simulink library "sub_lib_models"  (Simulink 4.00)
undefined symbols (not defined in the file or in its folder): vinf
libraries: lib_cosimulation x22
settings Model: LastModifiedBy=abrooker
settings Model: ModifiedComment=|
  | abrooker -- Thu May 02 17:18:54 2002 -- Version 1.26
  | fixed starter load level for non-cosim runs
settings Model: ModifiedHistory=|
  | abrooker -- Thu May 02 17:18:54 2002 -- Version 1.26
  | fixed starter load level for non-cosim runs
  | 
  | abrooker -- Wed Apr 24 09:14:19 2002 -- Version 1.25
  | 
  | 
  | abrooker -- Fri Apr 19 08:51:04 2002 -- Version 1.24
  | 
  | 
  | abrooker -- Fri Apr 19 08:49:53 2002 -- Version 1.23
  | 
  | 
  | mokeefe -- Thu Apr 18 08:41:06 2002 -- Version 1.22
  | saving the model:
  | o "without the model browser open"
  | o with only top-level screen visible
  | o with "fit to view" enabled
  | o with "status bar" off and "toolbar" off
  | o with "prompt to update model history with each save" on

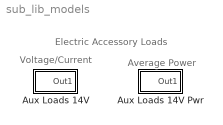
== system sub_lib_models ==
  note: Electric Accessory Loads
  note: Voltage/Current
  note: Average Power
  Aux Loads 14V : Subsystem
      settings: RTWFcnNameOpts=Auto  RTWFileNameOpts=Auto
  Aux Loads 14V Pwr : Subsystem
      settings: RTWFcnNameOpts=Auto  RTWFileNameOpts=Auto

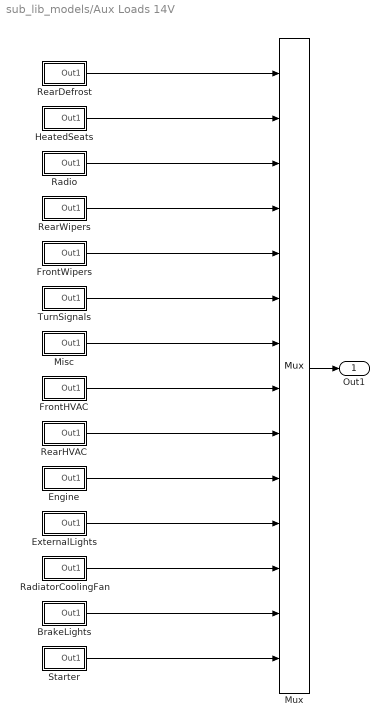
== system sub_lib_models/Aux Loads 14V ==
  BrakeLights : Subsystem
      settings: RTWFcnNameOpts=Auto  RTWFileNameOpts=Auto
  Engine : Subsystem
      settings: RTWFcnNameOpts=Auto  RTWFileNameOpts=Auto
  ExternalLights : Subsystem
      settings: RTWFcnNameOpts=Auto  RTWFileNameOpts=Auto
  FrontHVAC : Subsystem
      settings: RTWFcnNameOpts=Auto  RTWFileNameOpts=Auto
  FrontWipers : Subsystem
      settings: RTWFcnNameOpts=Auto  RTWFileNameOpts=Auto
  HeatedSeats : Subsystem
      settings: RTWFcnNameOpts=Auto  RTWFileNameOpts=Auto
  Misc : Subsystem
      settings: RTWFcnNameOpts=Auto  RTWFileNameOpts=Auto
  Mux : Mux  Inputs=[8 9 8 8 8 8 8 9 9 8 9 9 8 2]
      settings: DisplayOption=none
  RadiatorCoolingFan : Subsystem
      settings: RTWFcnNameOpts=Auto  RTWFileNameOpts=Auto
  Radio : Subsystem
      settings: RTWFcnNameOpts=Auto  RTWFileNameOpts=Auto
  RearDefrost : Subsystem
      settings: RTWFcnNameOpts=Auto  RTWFileNameOpts=Auto
  RearHVAC : Subsystem
      settings: RTWFcnNameOpts=Auto  RTWFileNameOpts=Auto
  RearWipers : Subsystem
      settings: RTWFcnNameOpts=Auto  RTWFileNameOpts=Auto
  Starter : Subsystem
      settings: RTWFcnNameOpts=Auto  RTWFileNameOpts=Auto
  TurnSignals : Subsystem
      settings: RTWFcnNameOpts=Auto  RTWFileNameOpts=Auto
  Out1 : Outport  Port=1
  wires:
  Starter/1(Out1) -> Mux/14
  BrakeLights/1(Out1) -> Mux/13
  RadiatorCoolingFan/1(Out1) -> Mux/12
  ExternalLights/1(Out1) -> Mux/11
  Engine/1(Out1) -> Mux/10
  RearHVAC/1(Out1) -> Mux/9
  FrontHVAC/1(Out1) -> Mux/8
  Misc/1(Out1) -> Mux/7
  TurnSignals/1(Out1) -> Mux/6
  FrontWipers/1(Out1) -> Mux/5
  RearWipers/1(Out1) -> Mux/4
  Radio/1(Out1) -> Mux/3
  HeatedSeats/1(Out1) -> Mux/2
  RearDefrost/1(Out1) -> Mux/1
  Mux/1 -> Out1/1

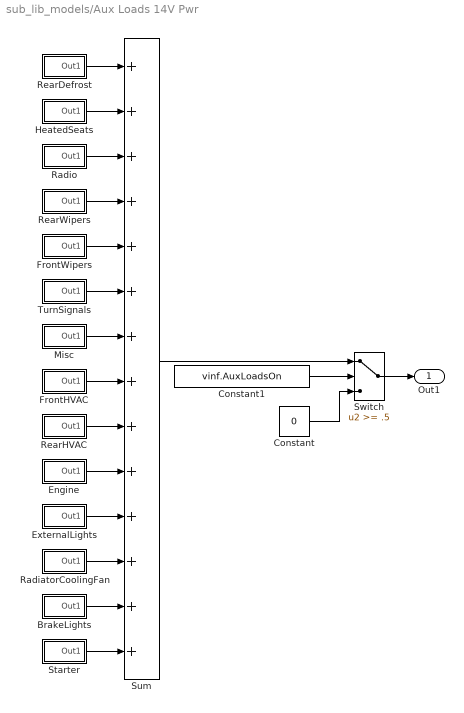
== system sub_lib_models/Aux Loads 14V Pwr ==
  BrakeLights : Subsystem
      settings: RTWFcnNameOpts=Auto  RTWFileNameOpts=Auto
  Constant : Constant  Value=0
  Constant1 : Constant  Value=vinf.AuxLoadsOn
  Engine : Subsystem
      settings: RTWFcnNameOpts=Auto  RTWFileNameOpts=Auto
  ExternalLights : Subsystem
      settings: RTWFcnNameOpts=Auto  RTWFileNameOpts=Auto
  FrontHVAC : Subsystem
      settings: RTWFcnNameOpts=Auto  RTWFileNameOpts=Auto
  FrontWipers : Subsystem
      settings: RTWFcnNameOpts=Auto  RTWFileNameOpts=Auto
  HeatedSeats : Subsystem
      settings: RTWFcnNameOpts=Auto  RTWFileNameOpts=Auto
  Misc : Subsystem
      settings: RTWFcnNameOpts=Auto  RTWFileNameOpts=Auto
  RadiatorCoolingFan : Subsystem
      settings: RTWFcnNameOpts=Auto  RTWFileNameOpts=Auto
  Radio : Subsystem
      settings: RTWFcnNameOpts=Auto  RTWFileNameOpts=Auto
  RearDefrost : Subsystem
      settings: RTWFcnNameOpts=Auto  RTWFileNameOpts=Auto
  RearHVAC : Subsystem
      settings: RTWFcnNameOpts=Auto  RTWFileNameOpts=Auto
  RearWipers : Subsystem
      settings: RTWFcnNameOpts=Auto  RTWFileNameOpts=Auto
  Starter : Subsystem
      settings: RTWFcnNameOpts=Auto  RTWFileNameOpts=Auto
  Sum : Sum  Inputs=++++++++++++++  SaturateOnIntegerOverflow=on
  Switch : Switch  Threshold=.5
  TurnSignals : Subsystem
      settings: RTWFcnNameOpts=Auto  RTWFileNameOpts=Auto
  Out1 : Outport  Port=1
  wires:
  Switch/1 -> Out1/1
  Sum/1 -> Switch/1
  Constant/1 -> Switch/3
  Constant1/1 -> Switch/2
  RearDefrost/1(Out1) -> Sum/1
  HeatedSeats/1(Out1) -> Sum/2
  Radio/1(Out1) -> Sum/3
  RearWipers/1(Out1) -> Sum/4
  FrontWipers/1(Out1) -> Sum/5
  TurnSignals/1(Out1) -> Sum/6
  Misc/1(Out1) -> Sum/7
  FrontHVAC/1(Out1) -> Sum/8
  RearHVAC/1(Out1) -> Sum/9
  Engine/1(Out1) -> Sum/10
  ExternalLights/1(Out1) -> Sum/11
  RadiatorCoolingFan/1(Out1) -> Sum/12
  BrakeLights/1(Out1) -> Sum/13
  Starter/1(Out1) -> Sum/14

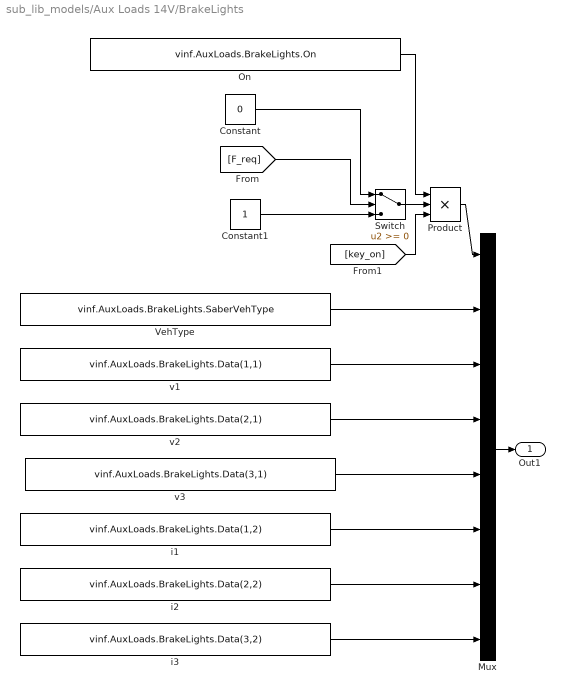
== system sub_lib_models/Aux Loads 14V/BrakeLights ==
  Constant : Constant  Value=0
  Constant1 : Constant  Value=1
  Mux : Mux  Inputs=8
  On : Constant  Value=vinf.AuxLoads.BrakeLights.On
  Product : Product  Inputs=3  Multiplication=Element-wise(.*)  SaturateOnIntegerOverflow=on
  Switch : Switch  Threshold=0
  VehType : Constant  Value=vinf.AuxLoads.BrakeLights.SaberVehType
  i1 : Constant  Value=vinf.AuxLoads.BrakeLights.Data(1,2)
  i2 : Constant  Value=vinf.AuxLoads.BrakeLights.Data(2,2)
  i3 : Constant  Value=vinf.AuxLoads.BrakeLights.Data(3,2)
  v1 : Constant  Value=vinf.AuxLoads.BrakeLights.Data(1,1)
  v2 : Constant  Value=vinf.AuxLoads.BrakeLights.Data(2,1)
  v3 : Constant  Value=vinf.AuxLoads.BrakeLights.Data(3,1)
  Out1 : Outport  Port=1
  wires:
  [key_on] -> Product/3
  VehType/1 -> Mux/2
  i3/1 -> Mux/8
  i2/1 -> Mux/7
  i1/1 -> Mux/6
  v3/1 -> Mux/5
  v2/1 -> Mux/4
  v1/1 -> Mux/3
  Mux/1 -> Out1/1
  On/1 -> Product/1
  Product/1 -> Mux/1
  Constant/1 -> Switch/1
  [F_req] -> Switch/2
  Constant1/1 -> Switch/3
  Switch/1 -> Product/2

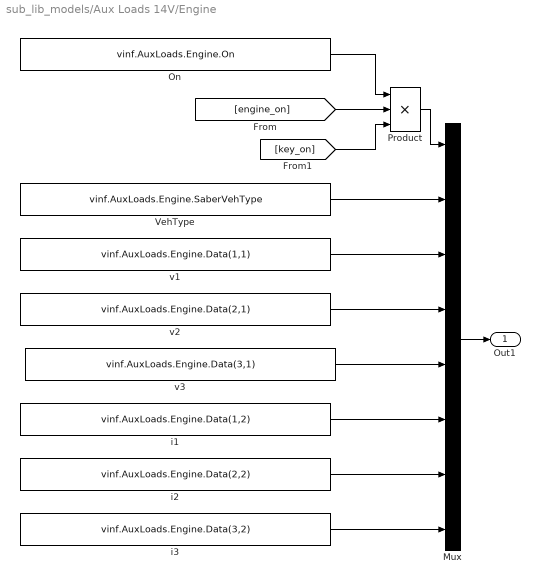
== system sub_lib_models/Aux Loads 14V/Engine ==
  Mux : Mux  Inputs=8
  On : Constant  Value=vinf.AuxLoads.Engine.On
  Product : Product  Inputs=3  Multiplication=Element-wise(.*)  SaturateOnIntegerOverflow=on
  VehType : Constant  Value=vinf.AuxLoads.Engine.SaberVehType
  i1 : Constant  Value=vinf.AuxLoads.Engine.Data(1,2)
  i2 : Constant  Value=vinf.AuxLoads.Engine.Data(2,2)
  i3 : Constant  Value=vinf.AuxLoads.Engine.Data(3,2)
  v1 : Constant  Value=vinf.AuxLoads.Engine.Data(1,1)
  v2 : Constant  Value=vinf.AuxLoads.Engine.Data(2,1)
  v3 : Constant  Value=vinf.AuxLoads.Engine.Data(3,1)
  Out1 : Outport  Port=1
  wires:
  [key_on] -> Product/3
  i3/1 -> Mux/8
  i2/1 -> Mux/7
  i1/1 -> Mux/6
  v3/1 -> Mux/5
  v2/1 -> Mux/4
  v1/1 -> Mux/3
  Mux/1 -> Out1/1
  On/1 -> Product/1
  [engine_on] -> Product/2
  Product/1 -> Mux/1
  VehType/1 -> Mux/2

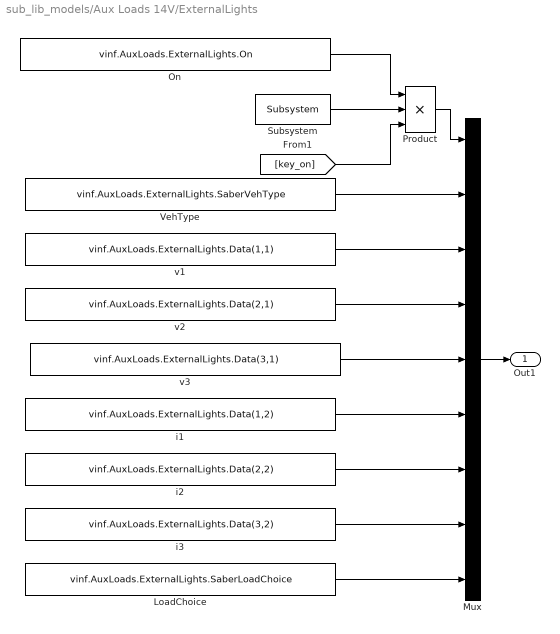
== system sub_lib_models/Aux Loads 14V/ExternalLights ==
  LoadChoice : Constant  Value=vinf.AuxLoads.ExternalLights.SaberLoadChoice
  Mux : Mux  Inputs=9
  On : Constant  Value=vinf.AuxLoads.ExternalLights.On
  Product : Product  Inputs=3  Multiplication=Element-wise(.*)  SaturateOnIntegerOverflow=on
  Subsystem : lib_cosimulation/Subsystem  ModelName='ExternalLights'
  VehType : Constant  Value=vinf.AuxLoads.ExternalLights.SaberVehType
  i1 : Constant  Value=vinf.AuxLoads.ExternalLights.Data(1,2)
  i2 : Constant  Value=vinf.AuxLoads.ExternalLights.Data(2,2)
  i3 : Constant  Value=vinf.AuxLoads.ExternalLights.Data(3,2)
  v1 : Constant  Value=vinf.AuxLoads.ExternalLights.Data(1,1)
  v2 : Constant  Value=vinf.AuxLoads.ExternalLights.Data(2,1)
  v3 : Constant  Value=vinf.AuxLoads.ExternalLights.Data(3,1)
  Out1 : Outport  Port=1
  wires:
  [key_on] -> Product/3
  LoadChoice/1 -> Mux/9
  i3/1 -> Mux/8
  i2/1 -> Mux/7
  i1/1 -> Mux/6
  v3/1 -> Mux/5
  v2/1 -> Mux/4
  v1/1 -> Mux/3
  VehType/1 -> Mux/2
  Mux/1 -> Out1/1
  On/1 -> Product/1
  Subsystem/1 -> Product/2
  Product/1 -> Mux/1

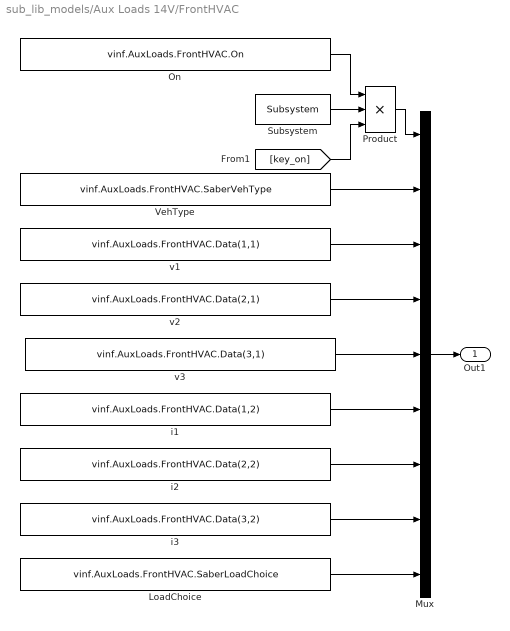
== system sub_lib_models/Aux Loads 14V/FrontHVAC ==
  LoadChoice : Constant  Value=vinf.AuxLoads.FrontHVAC.SaberLoadChoice
  Mux : Mux  Inputs=9
  On : Constant  Value=vinf.AuxLoads.FrontHVAC.On
  Product : Product  Inputs=3  Multiplication=Element-wise(.*)  SaturateOnIntegerOverflow=on
  Subsystem : lib_cosimulation/Subsystem  ModelName='FrontHVAC'
  VehType : Constant  Value=vinf.AuxLoads.FrontHVAC.SaberVehType
  i1 : Constant  Value=vinf.AuxLoads.FrontHVAC.Data(1,2)
  i2 : Constant  Value=vinf.AuxLoads.FrontHVAC.Data(2,2)
  i3 : Constant  Value=vinf.AuxLoads.FrontHVAC.Data(3,2)
  v1 : Constant  Value=vinf.AuxLoads.FrontHVAC.Data(1,1)
  v2 : Constant  Value=vinf.AuxLoads.FrontHVAC.Data(2,1)
  v3 : Constant  Value=vinf.AuxLoads.FrontHVAC.Data(3,1)
  Out1 : Outport  Port=1
  wires:
  [key_on] -> Product/3
  LoadChoice/1 -> Mux/9
  i3/1 -> Mux/8
  i2/1 -> Mux/7
  i1/1 -> Mux/6
  v3/1 -> Mux/5
  v2/1 -> Mux/4
  v1/1 -> Mux/3
  VehType/1 -> Mux/2
  Mux/1 -> Out1/1
  On/1 -> Product/1
  Subsystem/1 -> Product/2
  Product/1 -> Mux/1

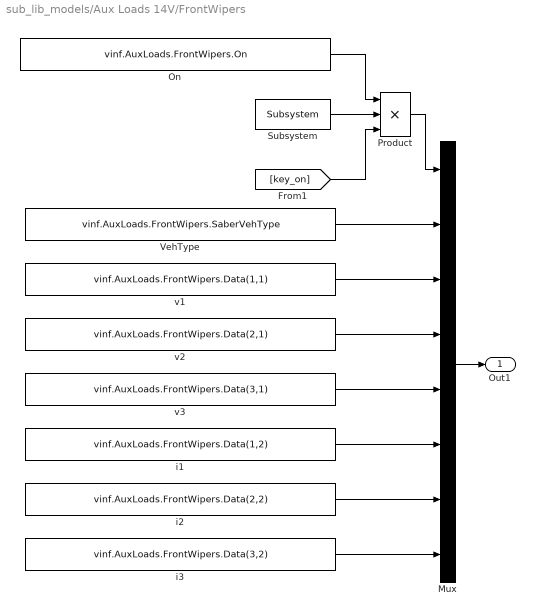
== system sub_lib_models/Aux Loads 14V/FrontWipers ==
  Mux : Mux  Inputs=8
  On : Constant  Value=vinf.AuxLoads.FrontWipers.On
  Product : Product  Inputs=3  Multiplication=Element-wise(.*)  SaturateOnIntegerOverflow=on
  Subsystem : lib_cosimulation/Subsystem  ModelName='FrontWipers'
  VehType : Constant  Value=vinf.AuxLoads.FrontWipers.SaberVehType
  i1 : Constant  Value=vinf.AuxLoads.FrontWipers.Data(1,2)
  i2 : Constant  Value=vinf.AuxLoads.FrontWipers.Data(2,2)
  i3 : Constant  Value=vinf.AuxLoads.FrontWipers.Data(3,2)
  v1 : Constant  Value=vinf.AuxLoads.FrontWipers.Data(1,1)
  v2 : Constant  Value=vinf.AuxLoads.FrontWipers.Data(2,1)
  v3 : Constant  Value=vinf.AuxLoads.FrontWipers.Data(3,1)
  Out1 : Outport  Port=1
  wires:
  [key_on] -> Product/3
  VehType/1 -> Mux/2
  i2/1 -> Mux/7
  i3/1 -> Mux/8
  i1/1 -> Mux/6
  v3/1 -> Mux/5
  v2/1 -> Mux/4
  v1/1 -> Mux/3
  Mux/1 -> Out1/1
  On/1 -> Product/1
  Subsystem/1 -> Product/2
  Product/1 -> Mux/1

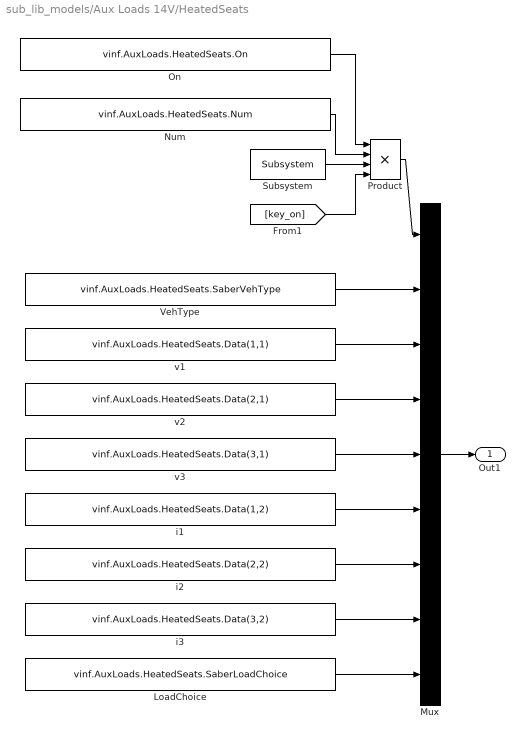
== system sub_lib_models/Aux Loads 14V/HeatedSeats ==
  LoadChoice : Constant  Value=vinf.AuxLoads.HeatedSeats.SaberLoadChoice
  Mux : Mux  Inputs=9
  Num : Constant  Value=vinf.AuxLoads.HeatedSeats.Num
  On : Constant  Value=vinf.AuxLoads.HeatedSeats.On
  Product : Product  Inputs=4  Multiplication=Element-wise(.*)  SaturateOnIntegerOverflow=on
  Subsystem : lib_cosimulation/Subsystem  ModelName='HeatedSeats'
  VehType : Constant  Value=vinf.AuxLoads.HeatedSeats.SaberVehType
  i1 : Constant  Value=vinf.AuxLoads.HeatedSeats.Data(1,2)
  i2 : Constant  Value=vinf.AuxLoads.HeatedSeats.Data(2,2)
  i3 : Constant  Value=vinf.AuxLoads.HeatedSeats.Data(3,2)
  v1 : Constant  Value=vinf.AuxLoads.HeatedSeats.Data(1,1)
  v2 : Constant  Value=vinf.AuxLoads.HeatedSeats.Data(2,1)
  v3 : Constant  Value=vinf.AuxLoads.HeatedSeats.Data(3,1)
  Out1 : Outport  Port=1
  wires:
  Product/1 -> Mux/1
  [key_on] -> Product/4
  Mux/1 -> Out1/1
  LoadChoice/1 -> Mux/9
  v1/1 -> Mux/3
  v2/1 -> Mux/4
  v3/1 -> Mux/5
  i1/1 -> Mux/6
  i2/1 -> Mux/7
  i3/1 -> Mux/8
  VehType/1 -> Mux/2
  On/1 -> Product/1
  Num/1 -> Product/2
  Subsystem/1 -> Product/3

== system sub_lib_models/Aux Loads 14V/Misc ==
  Mux : Mux  Inputs=8
  On : Constant  Value=vinf.AuxLoads.Misc.On
  Product : Product  Inputs=2  Multiplication=Element-wise(.*)  SaturateOnIntegerOverflow=on
  VehType : Constant  Value=vinf.AuxLoads.Misc.SaberVehType
  i1 : Constant  Value=vinf.AuxLoads.Misc.Data(1,2)
  i2 : Constant  Value=vinf.AuxLoads.Misc.Data(2,2)
  i3 : Constant  Value=vinf.AuxLoads.Misc.Data(3,2)
  v1 : Constant  Value=vinf.AuxLoads.Misc.Data(1,1)
  v2 : Constant  Value=vinf.AuxLoads.Misc.Data(2,1)
  v3 : Constant  Value=vinf.AuxLoads.Misc.Data(3,1)
  Out1 : Outport  Port=1
  wires:
  [key_on] -> Product/2
  On/1 -> Product/1
  Product/1 -> Mux/1
  VehType/1 -> Mux/2
  i3/1 -> Mux/8
  i2/1 -> Mux/7
  i1/1 -> Mux/6
  v3/1 -> Mux/5
  v2/1 -> Mux/4
  v1/1 -> Mux/3
  Mux/1 -> Out1/1

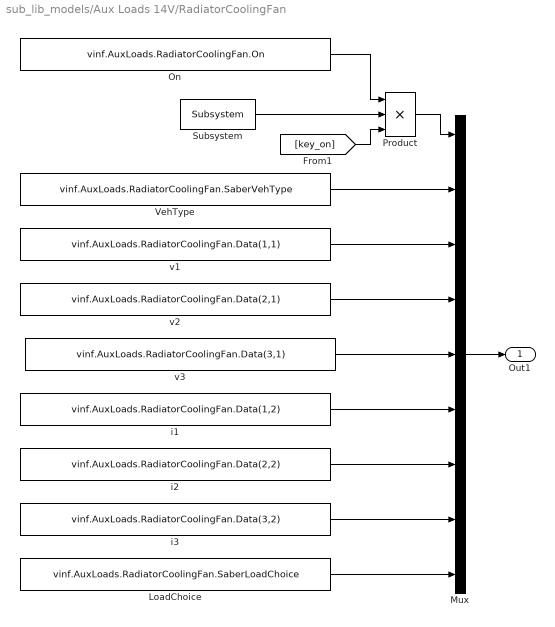
== system sub_lib_models/Aux Loads 14V/RadiatorCoolingFan ==
  LoadChoice : Constant  Value=vinf.AuxLoads.RadiatorCoolingFan.SaberLoadChoice
  Mux : Mux  Inputs=9
  On : Constant  Value=vinf.AuxLoads.RadiatorCoolingFan.On
  Product : Product  Inputs=3  Multiplication=Element-wise(.*)  SaturateOnIntegerOverflow=on
  Subsystem : lib_cosimulation/Subsystem  ModelName='RadiatorCoolingFan'
  VehType : Constant  Value=vinf.AuxLoads.RadiatorCoolingFan.SaberVehType
  i1 : Constant  Value=vinf.AuxLoads.RadiatorCoolingFan.Data(1,2)
  i2 : Constant  Value=vinf.AuxLoads.RadiatorCoolingFan.Data(2,2)
  i3 : Constant  Value=vinf.AuxLoads.RadiatorCoolingFan.Data(3,2)
  v1 : Constant  Value=vinf.AuxLoads.RadiatorCoolingFan.Data(1,1)
  v2 : Constant  Value=vinf.AuxLoads.RadiatorCoolingFan.Data(2,1)
  v3 : Constant  Value=vinf.AuxLoads.RadiatorCoolingFan.Data(3,1)
  Out1 : Outport  Port=1
  wires:
  [key_on] -> Product/3
  Mux/1 -> Out1/1
  LoadChoice/1 -> Mux/9
  i3/1 -> Mux/8
  i2/1 -> Mux/7
  i1/1 -> Mux/6
  v3/1 -> Mux/5
  v2/1 -> Mux/4
  v1/1 -> Mux/3
  VehType/1 -> Mux/2
  On/1 -> Product/1
  Subsystem/1 -> Product/2
  Product/1 -> Mux/1

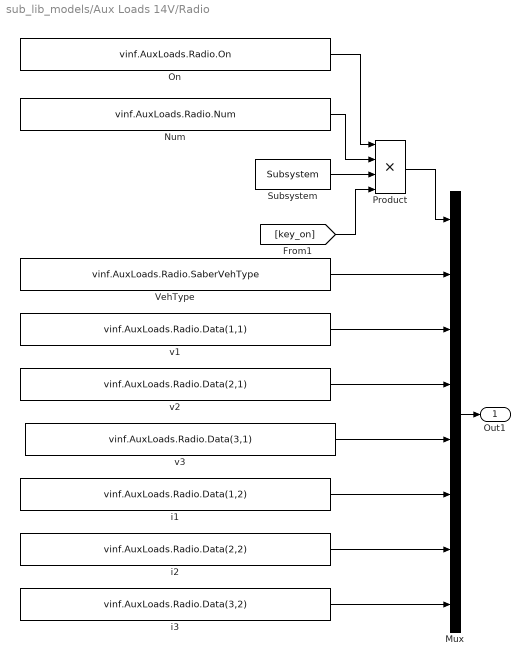
== system sub_lib_models/Aux Loads 14V/Radio ==
  Mux : Mux  Inputs=8
  Num : Constant  Value=vinf.AuxLoads.Radio.Num
  On : Constant  Value=vinf.AuxLoads.Radio.On
  Product : Product  Inputs=4  Multiplication=Element-wise(.*)  SaturateOnIntegerOverflow=on
  Subsystem : lib_cosimulation/Subsystem  ModelName='Radio'
  VehType : Constant  Value=vinf.AuxLoads.Radio.SaberVehType
  i1 : Constant  Value=vinf.AuxLoads.Radio.Data(1,2)
  i2 : Constant  Value=vinf.AuxLoads.Radio.Data(2,2)
  i3 : Constant  Value=vinf.AuxLoads.Radio.Data(3,2)
  v1 : Constant  Value=vinf.AuxLoads.Radio.Data(1,1)
  v2 : Constant  Value=vinf.AuxLoads.Radio.Data(2,1)
  v3 : Constant  Value=vinf.AuxLoads.Radio.Data(3,1)
  Out1 : Outport  Port=1
  wires:
  [key_on] -> Product/4
  i3/1 -> Mux/8
  i2/1 -> Mux/7
  i1/1 -> Mux/6
  v3/1 -> Mux/5
  v2/1 -> Mux/4
  v1/1 -> Mux/3
  VehType/1 -> Mux/2
  Mux/1 -> Out1/1
  On/1 -> Product/1
  Num/1 -> Product/2
  Subsystem/1 -> Product/3
  Product/1 -> Mux/1

== system sub_lib_models/Aux Loads 14V/RearDefrost ==
  Mux : Mux  Inputs=8
  On : Constant  Value=vinf.AuxLoads.RearDefrost.On
  Product : Product  Inputs=3  Multiplication=Element-wise(.*)  SaturateOnIntegerOverflow=on
  Subsystem : lib_cosimulation/Subsystem  ModelName='RearDefrost'
  VehType : Constant  Value=vinf.AuxLoads.RearDefrost.SaberVehType
  i1 : Constant  Value=vinf.AuxLoads.RearDefrost.Data(1,2)
  i2 : Constant  Value=vinf.AuxLoads.RearDefrost.Data(2,2)
  i3 : Constant  Value=vinf.AuxLoads.RearDefrost.Data(3,2)
  v1 : Constant  Value=vinf.AuxLoads.RearDefrost.Data(1,1)
  v2 : Constant  Value=vinf.AuxLoads.RearDefrost.Data(2,1)
  v3 : Constant  Value=vinf.AuxLoads.RearDefrost.Data(3,1)
  Out1 : Outport  Port=1
  wires:
  On/1 -> Product/1
  Subsystem/1 -> Product/2
  [key_on] -> Product/3
  Product/1 -> Mux/1
  VehType/1 -> Mux/2
  i3/1 -> Mux/8
  i2/1 -> Mux/7
  i1/1 -> Mux/6
  v3/1 -> Mux/5
  v2/1 -> Mux/4
  v1/1 -> Mux/3
  Mux/1 -> Out1/1

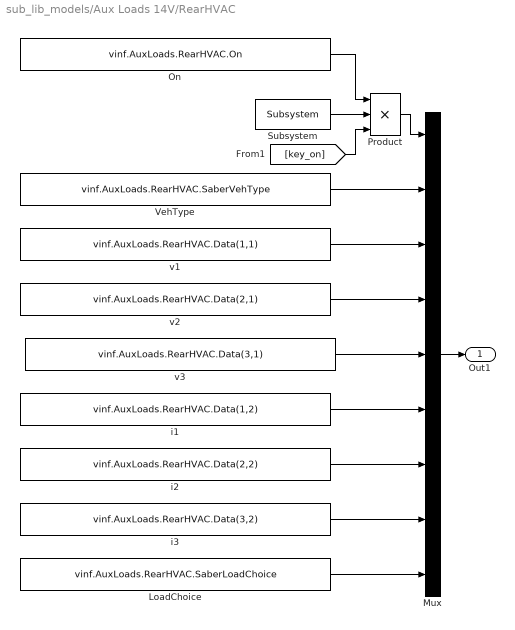
== system sub_lib_models/Aux Loads 14V/RearHVAC ==
  LoadChoice : Constant  Value=vinf.AuxLoads.RearHVAC.SaberLoadChoice
  Mux : Mux  Inputs=9
  On : Constant  Value=vinf.AuxLoads.RearHVAC.On
  Product : Product  Inputs=3  Multiplication=Element-wise(.*)  SaturateOnIntegerOverflow=on
  Subsystem : lib_cosimulation/Subsystem  ModelName='RearHVAC'
  VehType : Constant  Value=vinf.AuxLoads.RearHVAC.SaberVehType
  i1 : Constant  Value=vinf.AuxLoads.RearHVAC.Data(1,2)
  i2 : Constant  Value=vinf.AuxLoads.RearHVAC.Data(2,2)
  i3 : Constant  Value=vinf.AuxLoads.RearHVAC.Data(3,2)
  v1 : Constant  Value=vinf.AuxLoads.RearHVAC.Data(1,1)
  v2 : Constant  Value=vinf.AuxLoads.RearHVAC.Data(2,1)
  v3 : Constant  Value=vinf.AuxLoads.RearHVAC.Data(3,1)
  Out1 : Outport  Port=1
  wires:
  [key_on] -> Product/3
  LoadChoice/1 -> Mux/9
  i3/1 -> Mux/8
  i2/1 -> Mux/7
  i1/1 -> Mux/6
  v3/1 -> Mux/5
  v2/1 -> Mux/4
  v1/1 -> Mux/3
  Mux/1 -> Out1/1
  On/1 -> Product/1
  Subsystem/1 -> Product/2
  Product/1 -> Mux/1
  VehType/1 -> Mux/2

== system sub_lib_models/Aux Loads 14V/RearWipers ==
  Mux : Mux  Inputs=8
  On : Constant  Value=vinf.AuxLoads.RearWipers.On
  Product : Product  Inputs=3  Multiplication=Element-wise(.*)  SaturateOnIntegerOverflow=on
  Subsystem : lib_cosimulation/Subsystem  ModelName='RearWipers'
  VehType : Constant  Value=vinf.AuxLoads.RearWipers.SaberVehType
  i1 : Constant  Value=vinf.AuxLoads.RearWipers.Data(1,2)
  i2 : Constant  Value=vinf.AuxLoads.RearWipers.Data(2,2)
  i3 : Constant  Value=vinf.AuxLoads.RearWipers.Data(3,2)
  v1 : Constant  Value=vinf.AuxLoads.RearWipers.Data(1,1)
  v2 : Constant  Value=vinf.AuxLoads.RearWipers.Data(2,1)
  v3 : Constant  Value=vinf.AuxLoads.RearWipers.Data(3,1)
  Out1 : Outport  Port=1
  wires:
  [key_on] -> Product/3
  i3/1 -> Mux/8
  i2/1 -> Mux/7
  i1/1 -> Mux/6
  v3/1 -> Mux/5
  v2/1 -> Mux/4
  v1/1 -> Mux/3
  Mux/1 -> Out1/1
  On/1 -> Product/1
  Subsystem/1 -> Product/2
  Product/1 -> Mux/1
  VehType/1 -> Mux/2

== system sub_lib_models/Aux Loads 14V/Starter ==
  14 V : Constant  Value=vinf.AuxLoads.Starter.V14
  Hit  Crossing : HitCross  HitCrossingOffset=0  HitCrossingDirection=rising  ShowOutputPort=on
  Mux : Mux  Inputs=2
  On : Constant  Value=vinf.AuxLoads.Starter.On
  Product1 : Product  Inputs=4  Multiplication=Element-wise(.*)  SaturateOnIntegerOverflow=on
  Subsystem : lib_cosimulation/14V Load Control/Starter/Subsystem
      settings: RTWFcnNameOpts=Auto  RTWFileNameOpts=Auto
  starter_load (power) : Constant  Value=vinf.AuxLoads.Starter.Data
  Out1 : Outport  Port=1
  wires:
  Mux/1 -> Out1/1
  starter_load (power)/1 -> Mux/2
  14 V/1 -> Product1/2
  Subsystem/1 -> Product1/3
  Product1/1 -> Mux/1
  On/1 -> Product1/1
  [key_on] -> Product1/4
  [time] -> Subsystem/2
  [engine_on] -> Hit  Crossing/1
  Hit  Crossing/1 -> Subsystem/1

== system sub_lib_models/Aux Loads 14V/TurnSignals ==
  Mux : Mux  Inputs=8
  On : Constant  Value=vinf.AuxLoads.TurnSignals.On
  Product : Product  Inputs=3  Multiplication=Element-wise(.*)  SaturateOnIntegerOverflow=on
  Subsystem : lib_cosimulation/Subsystem  ModelName='TurnSignals'
  VehType : Constant  Value=vinf.AuxLoads.TurnSignals.SaberVehType
  i1 : Constant  Value=vinf.AuxLoads.TurnSignals.Data(1,2)
  i2 : Constant  Value=vinf.AuxLoads.TurnSignals.Data(2,2)
  i3 : Constant  Value=vinf.AuxLoads.TurnSignals.Data(3,2)
  v1 : Constant  Value=vinf.AuxLoads.TurnSignals.Data(1,1)
  v2 : Constant  Value=vinf.AuxLoads.TurnSignals.Data(2,1)
  v3 : Constant  Value=vinf.AuxLoads.TurnSignals.Data(3,1)
  Out1 : Outport  Port=1
  wires:
  [key_on] -> Product/3
  i3/1 -> Mux/8
  i2/1 -> Mux/7
  i1/1 -> Mux/6
  v3/1 -> Mux/5
  v2/1 -> Mux/4
  v1/1 -> Mux/3
  Mux/1 -> Out1/1
  On/1 -> Product/1
  Subsystem/1 -> Product/2
  Product/1 -> Mux/1
  VehType/1 -> Mux/2

== system sub_lib_models/Aux Loads 14V Pwr/BrakeLights ==
  Average Watts : Constant  Value=vinf.AuxLoads.BrakeLights.AverageWatts
  Constant : Constant  Value=0
  Constant1 : Constant  Value=1
  On : Constant  Value=vinf.AuxLoads.BrakeLights.On
  Product : Product  Inputs=4  Multiplication=Element-wise(.*)  SaturateOnIntegerOverflow=on
  Switch : Switch  Threshold=0
  Out1 : Outport  Port=1
  wires:
  Switch/1 -> Product/2
  On/1 -> Product/1
  [key_on] -> Product/3
  Average Watts/1 -> Product/4
  Constant1/1 -> Switch/3
  [F_req] -> Switch/2
  Constant/1 -> Switch/1
  Product/1 -> Out1/1

== system sub_lib_models/Aux Loads 14V Pwr/Engine ==
  Average Watts : Constant  Value=vinf.AuxLoads.Engine.AverageWatts
  Memory : Memory  X0=0  InheritSampleTime=off
      settings: RTWStateStorageClass=Auto
  On : Constant  Value=vinf.AuxLoads.Engine.On
  Product : Product  Inputs=4  Multiplication=Element-wise(.*)  SaturateOnIntegerOverflow=on
  Out1 : Outport  Port=1
  wires:
  Average Watts/1 -> Product/4
  Product/1 -> Out1/1
  On/1 -> Product/1
  [key_on] -> Product/3
  [engine_on] -> Memory/1
  Memory/1 -> Product/2

== system sub_lib_models/Aux Loads 14V Pwr/ExternalLights ==
  Average Watts : Constant  Value=vinf.AuxLoads.ExternalLights.AverageWatts
  On : Constant  Value=vinf.AuxLoads.ExternalLights.On
  Product : Product  Inputs=4  Multiplication=Element-wise(.*)  SaturateOnIntegerOverflow=on
  Subsystem : lib_cosimulation/Subsystem  ModelName='ExternalLights'
  Out1 : Outport  Port=1
  wires:
  Product/1 -> Out1/1
  Subsystem/1 -> Product/2
  On/1 -> Product/1
  [key_on] -> Product/3
  Average Watts/1 -> Product/4

== system sub_lib_models/Aux Loads 14V Pwr/FrontHVAC ==
  Average Watts : Constant  Value=vinf.AuxLoads.FrontHVAC.AverageWatts
  On : Constant  Value=vinf.AuxLoads.FrontHVAC.On
  Product : Product  Inputs=4  Multiplication=Element-wise(.*)  SaturateOnIntegerOverflow=on
  Subsystem : lib_cosimulation/Subsystem  ModelName='FrontHVAC'
  Out1 : Outport  Port=1
  wires:
  Product/1 -> Out1/1
  Subsystem/1 -> Product/2
  On/1 -> Product/1
  [key_on] -> Product/3
  Average Watts/1 -> Product/4

== system sub_lib_models/Aux Loads 14V Pwr/FrontWipers ==
  Average Watts : Constant  Value=vinf.AuxLoads.FrontWipers.AverageWatts
  On : Constant  Value=vinf.AuxLoads.FrontWipers.On
  Product : Product  Inputs=4  Multiplication=Element-wise(.*)  SaturateOnIntegerOverflow=on
  Subsystem : lib_cosimulation/Subsystem  ModelName='FrontWipers'
  Out1 : Outport  Port=1
  wires:
  Product/1 -> Out1/1
  Subsystem/1 -> Product/2
  On/1 -> Product/1
  [key_on] -> Product/3
  Average Watts/1 -> Product/4

== system sub_lib_models/Aux Loads 14V Pwr/HeatedSeats ==
  Average Watts : Constant  Value=vinf.AuxLoads.HeatedSeats.AverageWatts
  Num : Constant  Value=vinf.AuxLoads.HeatedSeats.Num
  On : Constant  Value=vinf.AuxLoads.HeatedSeats.On
  Product : Product  Inputs=5  Multiplication=Element-wise(.*)  SaturateOnIntegerOverflow=on
  Subsystem : lib_cosimulation/Subsystem  ModelName='HeatedSeats'
  Out1 : Outport  Port=1
  wires:
  Num/1 -> Product/2
  On/1 -> Product/1
  [key_on] -> Product/4
  Average Watts/1 -> Product/5
  Product/1 -> Out1/1
  Subsystem/1 -> Product/3

== system sub_lib_models/Aux Loads 14V Pwr/Misc ==
  Average Watts : Constant  Value=vinf.AuxLoads.Misc.AverageWatts
  On : Constant  Value=vinf.AuxLoads.Misc.On
  Product : Product  Inputs=3  Multiplication=Element-wise(.*)  SaturateOnIntegerOverflow=on
  Out1 : Outport  Port=1
  wires:
  Product/1 -> Out1/1
  On/1 -> Product/1
  [key_on] -> Product/2
  Average Watts/1 -> Product/3

== system sub_lib_models/Aux Loads 14V Pwr/RadiatorCoolingFan ==
  Average Watts : Constant  Value=vinf.AuxLoads.RadiatorCoolingFan.AverageWatts
  On : Constant  Value=vinf.AuxLoads.RadiatorCoolingFan.On
  Product : Product  Inputs=4  Multiplication=Element-wise(.*)  SaturateOnIntegerOverflow=on
  Subsystem : lib_cosimulation/Subsystem  ModelName='RadiatorCoolingFan'
  Out1 : Outport  Port=1
  wires:
  Product/1 -> Out1/1
  Subsystem/1 -> Product/2
  On/1 -> Product/1
  [key_on] -> Product/3
  Average Watts/1 -> Product/4

== system sub_lib_models/Aux Loads 14V Pwr/Radio ==
  Average Watts : Constant  Value=vinf.AuxLoads.Radio.AverageWatts
  Num : Constant  Value=vinf.AuxLoads.Radio.Num
  On : Constant  Value=vinf.AuxLoads.Radio.On
  Product : Product  Inputs=5  Multiplication=Element-wise(.*)  SaturateOnIntegerOverflow=on
  Subsystem : lib_cosimulation/Subsystem  ModelName='Radio'
  Out1 : Outport  Port=1
  wires:
  Product/1 -> Out1/1
  Num/1 -> Product/2
  On/1 -> Product/1
  [key_on] -> Product/4
  Average Watts/1 -> Product/5
  Subsystem/1 -> Product/3

== system sub_lib_models/Aux Loads 14V Pwr/RearDefrost ==
  Average Watts : Constant  Value=vinf.AuxLoads.RearDefrost.AverageWatts
  On : Constant  Value=vinf.AuxLoads.RearDefrost.On
  Product : Product  Inputs=4  Multiplication=Element-wise(.*)  SaturateOnIntegerOverflow=on
  Subsystem : lib_cosimulation/Subsystem  ModelName='RearDefrost'
  Out1 : Outport  Port=1
  wires:
  Product/1 -> Out1/1
  [key_on] -> Product/3
  On/1 -> Product/1
  Average Watts/1 -> Product/4
  Subsystem/1 -> Product/2

== system sub_lib_models/Aux Loads 14V Pwr/RearHVAC ==
  Average Watts : Constant  Value=vinf.AuxLoads.RearHVAC.AverageWatts
  On : Constant  Value=vinf.AuxLoads.RearHVAC.On
  Product : Product  Inputs=4  Multiplication=Element-wise(.*)  SaturateOnIntegerOverflow=on
  Subsystem : lib_cosimulation/Subsystem  ModelName='RearHVAC'
  Out1 : Outport  Port=1
  wires:
  Product/1 -> Out1/1
  Subsystem/1 -> Product/2
  On/1 -> Product/1
  [key_on] -> Product/3
  Average Watts/1 -> Product/4

== system sub_lib_models/Aux Loads 14V Pwr/RearWipers ==
  Average Watts : Constant  Value=vinf.AuxLoads.RearWipers.AverageWatts
  On : Constant  Value=vinf.AuxLoads.RearWipers.On
  Product : Product  Inputs=4  Multiplication=Element-wise(.*)  SaturateOnIntegerOverflow=on
  Subsystem : lib_cosimulation/Subsystem  ModelName='RearWipers'
  Out1 : Outport  Port=1
  wires:
  Product/1 -> Out1/1
  Subsystem/1 -> Product/2
  On/1 -> Product/1
  [key_on] -> Product/3
  Average Watts/1 -> Product/4

== system sub_lib_models/Aux Loads 14V Pwr/Starter ==
  Product1 : Product  Inputs=2  Multiplication=Element-wise(.*)  SaturateOnIntegerOverflow=on
  Starter : lib_cosimulation/14V Load Control/Starter
      settings: RTWFcnNameOpts=Auto  RTWFileNameOpts=Auto
  starter_load (power) : Constant  Value=vinf.AuxLoads.Starter.AverageWatts
  Out1 : Outport  Port=1
  wires:
  Product1/1 -> Out1/1
  starter_load (power)/1 -> Product1/2
  Starter/1 -> Product1/1

== system sub_lib_models/Aux Loads 14V Pwr/TurnSignals ==
  Average Watts : Constant  Value=vinf.AuxLoads.TurnSignals.AverageWatts
  On : Constant  Value=vinf.AuxLoads.TurnSignals.On
  Product : Product  Inputs=4  Multiplication=Element-wise(.*)  SaturateOnIntegerOverflow=on
  Subsystem : lib_cosimulation/Subsystem  ModelName='TurnSignals'
  Out1 : Outport  Port=1
  wires:
  Product/1 -> Out1/1
  Subsystem/1 -> Product/2
  On/1 -> Product/1
  [key_on] -> Product/3
  Average Watts/1 -> Product/4
